simulink model "extra_blocks"  (Simulink 7.4)
settings: Solver=FixedStepDiscrete  StartTime=0.0  StopTime=10.0  RelTol=1e-3
undefined symbols (not defined in the file or in its folder): Ax, Ay, Az, DiscIntNeverNeededParam, lenA, sys1d, vargz
libraries: simulink x8, dspsigops x1, commanapbnd3 x1, instrumentlib x1
(part 2 of 2)

== matlab function Equivalent to 2nd order transfer function w/ 1 zero/constants ==
  data: d output double; c output double; b output double; a output double
function [d, c, b, a] = f

%#eml

% Plant: G(s) = ds + c/(s^2 + as + b)

% zeta = sqrt(2)/2;
% om = 1.4;   % from 1.4 to 1.0
% K = 1;
% a = 1;  % small

% num = [K*(om^2)/a K*om^2];   % (om^2/a)(s+a)
% den = [1 2*zeta*om om^2];
% sysout = tf(num, den);

% num = [0.007825 - 0.007793]
% den = [1 -1.992 0.9921]

% Transfer function:     (K=1,a=1 - iMose can do this plant)
% 0.007825 z - 0.007793
% ----------------------
% z^2 - 1.992 z + 0.9921

% Continuous coefficients
% b = om^2;
% a = 2*zeta*om;
% c = om^2;
% d = (om^2)/a;

% Discrete coefficients
b = 0.9921;
a = -1.992;
c = -0.007793;
d = 0.007825;

== matlab function Equivalent to 2nd order transfer function w/ 1 zero/discrete_integrator ==
  data: out output double; in input double; in_prev input double; in_sum_prev input double; in_sum output double; event input double
function [out, in_sum] = f(in, in_prev, in_sum_prev, event)

%#eml

Ki = 1;

if (event == 4)
    % Sum the input
    in_increment = in - in_prev;
    in_sum = in_sum_prev + in_increment;
    out = Ki*(in_sum);
else
    % Reset
    in_sum = 0;
    out = 0;
end

== matlab function Equivalent to 2nd order transfer function w/ 1 zero/discrete_integrator1 ==
  data: out output double; in input double; in_prev input double; in_sum_prev input double; in_sum output double; event input double
function [out, in_sum] = f(in, in_prev, in_sum_prev, event)

%#eml

Ki = 1;

if (event == 4)
    % Sum the input
    in_increment = in - in_prev;
    in_sum = in_sum_prev + in_increment;
    out = Ki*(in_sum);
else
    % Reset
    in_sum = 0;
    out = 0;
end

== matlab function Equivalent to 2nd order transfer function w/ 1 zero/discrete_integrator2 ==
  data: out output double; in input double; in_prev input double; in_sum_prev input double; in_sum output double; event input double
function [out, in_sum] = f(in, in_prev, in_sum_prev, event)

%#eml

Ki = 1;

if (event == 4)
    % Sum the input
    in_increment = in - in_prev;
    in_sum = in_sum_prev + in_increment;
    out = Ki*(in_sum);
else
    % Reset
    in_sum = 0;
    out = 0;
end

== matlab function Butterworth filter-lowpass 0.01Hz: Equivalent to 2nd order transfer function w/ 2 zeros/constants ==
  data: e output double; d output double; c output double; b output double; a output double
function [e, d, c, b, a] = f

%#eml

% Plant: G(s) = es^2 + ds + c/(s^2 + as + b)

% num = [0.0002414 0.0004827 0.0002414];
% den = [1 -1.9556 0.9565];
% Ts = 0.004;
% sysout_dis = tf(num, den, Ts);
% sysout_con = d2c(sysout_dis)
% 
% Transfer function:
% 0.0002414 s^2 + 0.1225 s + 61.7
% -------------------------------
%      s^2 + 11.12 s + 57.51

% Continuous coefficients
% b = 57.51;
% a = 11.12;
% c = 61.7;
% d = 0.1225;
% e = 0.0002414;

% Discrete coefficients
b = 0.9565;
a = -1.9556;
c = 0.0002414;
d = 0.0004827;
e = 0.0002414;

== matlab function Butterworth filter-lowpass 0.01Hz: Equivalent to 2nd order transfer function w/ 2 zeros/discrete_integrator ==
  data: out output double; in input double; in_prev input double; in_sum_prev input double; in_sum output double; event input double
function [out, in_sum] = f(in, in_prev, in_sum_prev, event)

%#eml

Ki = 1;

if (event == 4)
    % Sum the input
    in_increment = in - in_prev;
    in_sum = in_sum_prev + in_increment;
    out = Ki*(in_sum);
else
    % Reset
    in_sum = 0;
    out = 0;
end

== matlab function Butterworth filter-lowpass 0.01Hz: Equivalent to 2nd order transfer function w/ 2 zeros/discrete_integrator1 ==
  data: out output double; in input double; in_prev input double; in_sum_prev input double; in_sum output double; event input double
function [out, in_sum] = f(in, in_prev, in_sum_prev, event)

%#eml

Ki = 1;

if (event == 4)
    % Sum the input
    in_increment = in - in_prev;
    in_sum = in_sum_prev + in_increment;
    out = Ki*(in_sum);
else
    % Reset
    in_sum = 0;
    out = 0;
end

== matlab function Butterworth filter-lowpass 0.01Hz: Equivalent to 2nd order transfer function w/ 2 zeros/discrete_integrator2 ==
  data: out output double; in input double; in_prev input double; in_sum_prev input double; in_sum output double; event input double
function [out, in_sum] = f(in, in_prev, in_sum_prev, event)

%#eml

Ki = 1;

if (event == 4)
    % Sum the input
    in_increment = in - in_prev;
    in_sum = in_sum_prev + in_increment;
    out = Ki*(in_sum);
else
    % Reset
    in_sum = 0;
    out = 0;
end

== matlab function Butterworth filter-lowpass 0.01Hz: Equivalent to 2nd order transfer function w/ 2 zeros/discrete_integrator3 ==
  data: out output double; in input double; in_prev input double; in_sum_prev input double; in_sum output double; event input double
function [out, in_sum] = f(in, in_prev, in_sum_prev, event)

%#eml

Ki = 1;

if (event == 4)
    % Sum the input
    in_increment = in - in_prev;
    in_sum = in_sum_prev + in_increment;
    out = Ki*(in_sum);
else
    % Reset
    in_sum = 0;
    out = 0;
end

== matlab function Butterworth filter-lowpass 0.01Hz: Equivalent to 2nd order transfer function w/ 2 zeros1/constants ==
  data: e output double; d output double; c output double; b output double; a output double
function [e, d, c, b, a] = f

%#eml

% Plant: G(s) = es^2 + ds + c/(s^2 + as + b)

% num = [0.0002414 0.0004827 0.0002414];
% den = [1 -1.9556 0.9565];
% Ts = 0.004;
% sysout_dis = tf(num, den, Ts);
% sysout_con = d2c(sysout_dis)
% 
% Transfer function:
% 0.0002414 s^2 + 0.1225 s + 61.7
% -------------------------------
%      s^2 + 11.12 s + 57.51

% Continuous coefficients
% b = 57.51;
% a = 11.12;
% c = 61.7;
% d = 0.1225;
% e = 0.0002414;

% Discrete coefficients
b = 0.9565;
a = -1.9556;
c = 0.0002414;
d = 0.0004827;
e = 0.0002414;

== matlab function Butterworth filter-lowpass 0.01Hz: Equivalent to 2nd order transfer function w/ 2 zeros1/discrete_integrator ==
  data: out output double; in input double; in_prev input double; in_sum_prev input double; in_sum output double; event input double
function [out, in_sum] = f(in, in_prev, in_sum_prev, event)

%#eml

Ki = 1;

if (event == 4)
    % Sum the input
    in_increment = in - in_prev;
    in_sum = in_sum_prev + in_increment;
    out = Ki*(in_sum);
else
    % Reset
    in_sum = 0;
    out = 0;
end

== matlab function Butterworth filter-lowpass 0.01Hz: Equivalent to 2nd order transfer function w/ 2 zeros1/discrete_integrator1 ==
  data: out output double; in input double; in_prev input double; in_sum_prev input double; in_sum output double; event input double
function [out, in_sum] = f(in, in_prev, in_sum_prev, event)

%#eml

Ki = 1;

if (event == 4)
    % Sum the input
    in_increment = in - in_prev;
    in_sum = in_sum_prev + in_increment;
    out = Ki*(in_sum);
else
    % Reset
    in_sum = 0;
    out = 0;
end

== matlab function Butterworth filter-lowpass 0.01Hz: Equivalent to 2nd order transfer function w/ 2 zeros1/discrete_integrator2 ==
  data: out output double; in input double; in_prev input double; in_sum_prev input double; in_sum output double; event input double
function [out, in_sum] = f(in, in_prev, in_sum_prev, event)

%#eml

Ki = 1;

if (event == 4)
    % Sum the input
    in_increment = in - in_prev;
    in_sum = in_sum_prev + in_increment;
    out = Ki*(in_sum);
else
    % Reset
    in_sum = 0;
    out = 0;
end

== matlab function Butterworth filter-lowpass 0.01Hz: Equivalent to 2nd order transfer function w/ 2 zeros1/discrete_integrator3 ==
  data: out output double; in input double; in_prev input double; in_sum_prev input double; in_sum output double; event input double
function [out, in_sum] = f(in, in_prev, in_sum_prev, event)

%#eml

Ki = 1;

if (event == 4)
    % Sum the input
    in_increment = in - in_prev;
    in_sum = in_sum_prev + in_increment;
    out = Ki*(in_sum);
else
    % Reset
    in_sum = 0;
    out = 0;
end

== matlab function Equivalent to 2nd order transfer function/constants ==
  data: d output double; c output double; b output double; a output double
function [d, c, b, a] = f

%#eml

% Plant: G(s) = ds + c/(s^2 + as + b)

% -----------------------
% zeta = sqrt(2)/2;
% om = 1.4;   % from 1.4 to 1.0
% K = 1;
% a = 1;  % small

% num = [K*(om^2)/a K*om^2];   % (om^2/a)(s+a)
% den = [1 2*zeta*om om^2];
% sysout = tf(num, den);

% num = [0.007825 - 0.007793]
% den = [1 -1.992 0.9921]

% Transfer function:     (K=1,a=1 - iMose can do this plant)
% 0.007825 z - 0.007793
% ----------------------
% z^2 - 1.992 z + 0.9921
% -------> large response signal
% -----------------------

% -----------------------
% zeta = sqrt(2)/2;
% om = 1.4;   % from 1.4 to 1.0
% K = 0.5;
% a = 1;  % small
% num = [K*(om^2)/a K*om^2];   % (om^2/a)(s+a)
% den = [1 2*zeta*om om^2];
% sysout = tf(num, den);
% Ts = 0.004;
% c2d(sysout, Ts)

% Transfer function:
% 0.003912 z - 0.003897
% ----------------------
% z^2 - 1.992 z + 0.9921
%  
% Sampling time: 0.004
% -----------------------


% Discrete coefficients
b = 0.09921;
a = -0.1992;
c = -0.4793;
d = 0.4825;

== matlab function Equivalent to 2nd order transfer function/discrete_integrator ==
  data: out output double; in input double; in_prev input double; in_sum_prev input double; in_sum output double; event input double
function [out, in_sum] = f(in, in_prev, in_sum_prev, event)

%#eml

Ki = 1;

if (event == 4)
    % Sum the input
    in_increment = in - in_prev;
    in_sum = in_sum_prev + in_increment;
    out = Ki*(in_sum);
else
    % Reset
    in_sum = 0;
    out = 0;
end

== matlab function Equivalent to 2nd order transfer function/discrete_integrator1 ==
  data: out output double; in input double; in_prev input double; in_sum_prev input double; in_sum output double; event input double
function [out, in_sum] = f(in, in_prev, in_sum_prev, event)

%#eml

Ki = 1;

if (event == 4)
    % Sum the input
    in_increment = in - in_prev;
    in_sum = in_sum_prev + in_increment;
    out = Ki*(in_sum);
else
    % Reset
    in_sum = 0;
    out = 0;
end

== matlab function Equivalent to 2nd order transfer function/discrete_integrator2 ==
  data: out output double; in input double; in_prev input double; in_sum_prev input double; in_sum output double; event input double
function [out, in_sum] = f(in, in_prev, in_sum_prev, event)

%#eml

Ki = 1;

if (event == 4)
    % Sum the input
    in_increment = in - in_prev;
    in_sum = in_sum_prev + in_increment;
    out = Ki*(in_sum);
else
    % Reset
    in_sum = 0;
    out = 0;
end

== matlab function get max2 ==
  data: x input double; max_x output double; max_xprev input double
function max_x = f(x, max_xprev)

%#eml

%if (event > 1)

    max_x1 = max(abs(x(1,1))); % want max deviation from 0
    if max_x1 < max_xprev(1,1)
        max_x1 = max_xprev(1,1);
    end
    
    max_x2 = max(abs(x(2,1))); % want max deviation from 0
    if max_x2 < max_xprev(2,1)
        max_x2 = max_xprev(2,1);
    end
    
    max_x3 = max(abs(x(3,1))); % want max deviation from 0
    if max_x3 < max_xprev(3,1)
        max_x3 = max_xprev(3,1);
    end
    
    max_x4 = max(abs(x(4,1))); % want max deviation from 0
    if max_x4 < max_xprev(4,1)
        max_x4 = max_xprev(4,1);
    end
    
    max_x5 = max(abs(x(5,1))); % want max deviation from 0
    if max_x5 < max_xprev(5,1)
        max_x5 = max_xprev(5,1);
    end
    
    max_x6 = max(abs(x(6,1))); % want max deviation from 0
    if max_x6 < max_xprev(6,1)
        max_x6 = max_xprev(6,1);
    end
    

max_x = [max_x1; max_x2; max_x3; max_x4; max_x5; max_x6];
